simulink model "HW9"  (R2023b)
settings: Solver=FixedStepAuto  StartTime=0.0  StopTime=0.5  FixedStep=0.01  RelTol=1e-3
libraries: simulink_extras x3, sharedtransform x1, uavutilslib x1
settings Model: Creator=Bw Jiang  LastModifiedBy=Bw Jiang

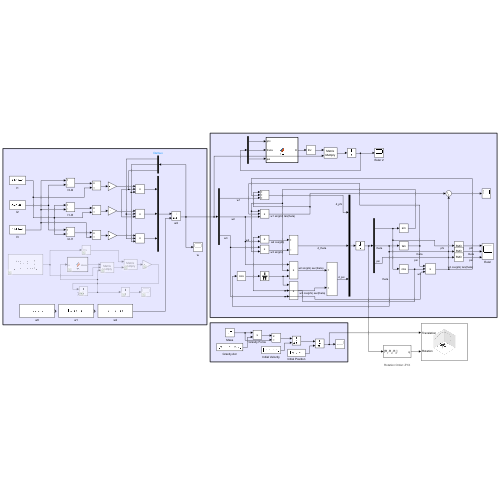
[thumbnail: Simulink's stored preview of the top-level diagram]
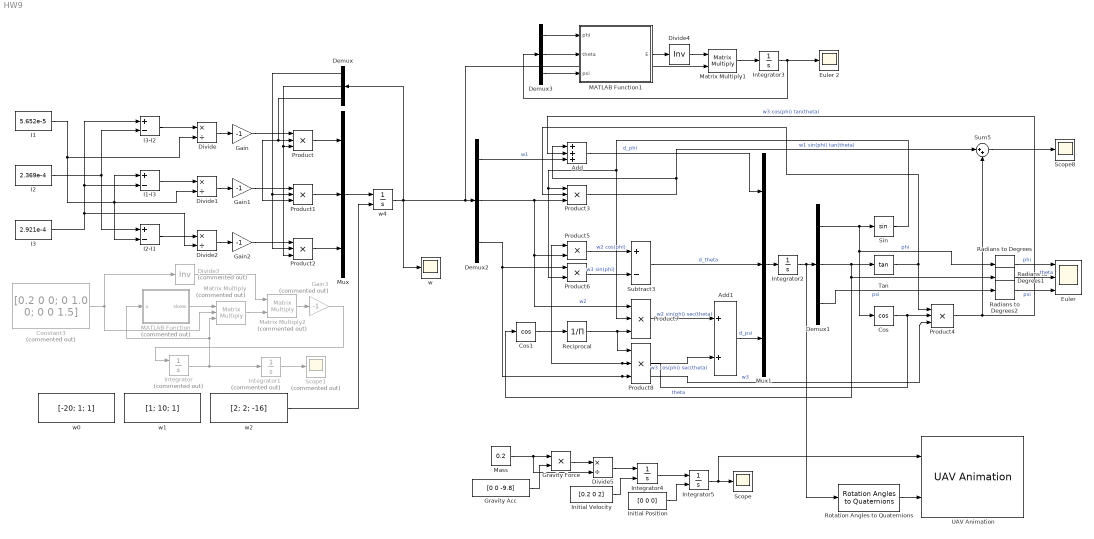
== system HW9 ==
  Add : Sum  Inputs=+++
  Add1 : Sum
  Constant3 : Constant  Commented=on  Value=[0.2 0 0; 0 1.0 0; 0 0 1.5]
  Cos : Trigonometry  Operator=cos
  Cos1 : Trigonometry  Operator=cos
  Demux{,1..3} (4 alike) : Demux  Outputs=3
  Divide{,1..2,5} (4 alike) : Product  Inputs=*/
  Divide3 : Product  Commented=on  Inputs=/  Multiplication=Matrix(*)
  Divide4 : Product  Inputs=/  Multiplication=Matrix(*)
  Euler : Scope  NumInputPorts=3
  Euler 2 : Scope
  Gain : Gain  Gain=-1
  Gain1 : Gain  Gain=-1
  Gain2 : Gain  Gain=-1
  Gain3 : Gain  Commented=on  Gain=-1
  Gravity Acc : Constant  Value=[0 0 -9.8]
  Gravity Force : Product
  I1 : Constant  Value=5.652e-5
  I1-I3 : Sum  Inputs=+-
  I2 : Constant  Value=2.369e-4
  I2-I1 : Sum  Inputs=+-
  I3 : Constant  Value=2.921e-4
  I3-I2 : Sum  Inputs=+-
  Initial Position : Constant  Value=[0 0 0]
  Initial Velocity : Constant  Value=[0.2 0 2]
  Integrator : Integrator  Commented=on  InitialConditionSource=external
  Integrator1 : Integrator  Commented=on
  Integrator2 : Integrator
  Integrator3 : Integrator
  Integrator4 : Integrator  InitialConditionSource=external
  Integrator5 : Integrator  InitialConditionSource=external
  MATLAB Function : MATLAB Function  Commented=on  TreatAsAtomicUnit=on
  MATLAB Function1 : MATLAB Function  TreatAsAtomicUnit=on
  Mass : Constant  Value=0.2
  Matrix Multiply : Product  Commented=on  Inputs=3  Multiplication=Matrix(*)
  Matrix Multiply1 : Product  Multiplication=Matrix(*)
  Matrix Multiply2 : Product  Commented=on  Multiplication=Matrix(*)
  Mux : Mux  Inputs=3
  Mux1 : Mux  Inputs=3
  Product{,1..4,7..8} (7 alike) : Product  Inputs=3
  Product5 : Product
  Product6 : Product
  Radians to Degrees : simulink_extras/Transformations/Radians to Degrees
  Radians to Degrees1 : simulink_extras/Transformations/Radians to Degrees
  Radians to Degrees2 : simulink_extras/Transformations/Radians to Degrees
  Reciprocal : Product  Inputs=/
  Rotation Angles to Quaternions : sharedtransform/Rotation Angles to Quaternions  rotationOrder=ZYX  aMode=aMode
  Scope : Scope
  Scope1 : Scope  Commented=on
  Scope8 : Scope
  Sin : Trigonometry
  Subtract3 : Sum  Inputs=+-
  Sum5 : Sum  Inputs=|++
  Tan : Trigonometry  Operator=tan
  UAV Animation : uavutilslib/UAV Animation  UAVType=FixedWing  UAVSize=0.1  InertialZDirection=Up  SampleTime=-1
  w : Scope
  w0 : Constant  Value=[-20; 1; 1]
  w1 : Constant  Value=[1; 10; 1]
  w2 : Constant  Value=[2; 2; -16]
  w4 : Integrator  InitialConditionSource=external
  wires:
  I3/1 -> Divide2/2, I3-I2/1, I1-I3/2
  I2/1 -> I2-I1/1, I3-I2/2
  I1/1 -> Divide1/2, I2-I1/2, I1-I3/1, Divide/2
  I3-I2/1 -> Divide/1
  I1-I3/1 -> Divide1/1
  I2-I1/1 -> Divide2/1
  Divide/1 -> Gain/1
  Divide2/1 -> Gain2/1
  Divide1/1 -> Gain1/1
  Gain/1 -> Product/1
  Gain1/1 -> Product1/1
  Product1/1 -> Mux/2
  Gain2/1 -> Product2/1
  Product2/1 -> Mux/3
  Product/1 -> Mux/1
  Constant3/1 -> Divide3/1, Matrix Multiply/2
  w2/1 -> w4/2
  Integrator/1 -> Integrator1/1, Matrix Multiply/3, MATLAB Function/1(u)
  MATLAB Function/1(skew) -> Matrix Multiply/1
  Divide3/1 -> Matrix Multiply2/1
  Matrix Multiply/1 -> Matrix Multiply2/2
  Matrix Multiply2/1 -> Gain3/1
  Gain3/1 -> Integrator/1
  Integrator1/1 -> Scope1/1
  Subtract3/1 -> Mux1/2  "d_theta"
  Demux1/3 -> Radians to Degrees2/1  "psi"
  Demux1/2 -> Tan/1, Cos1/1, Radians to Degrees1/1  "theta"
  Product3/1 -> Sum5/1, Add/1  "w1 sin(phi) tan(theta)"
  Product8/1 -> Add1/2  "w3 cos(phi) sec(theta)"
  Demux2/3 -> Product6/1, Product8/3, Product4/3  "w3"
  Add1/1 -> Mux1/3  "d_psi"
  Sum5/1 -> Scope8/1
  Product7/1 -> Add1/1  "w2 sin(phi) sec(theta)"
  Reciprocal/1 -> Product7/3, Product8/1
  Product5/1 -> Subtract3/1  "w2 cos(phi)"
  Cos1/1 -> Reciprocal/1
  Cos/1 -> Product4/2, Product5/1, Product8/2
  Demux1/1 -> Sin/1, Radians to Degrees/1, Cos/1  "phi"
  Tan/1 -> Product4/1, Product3/2
  Product4/1 -> Add/2, Sum5/2  "w3 cos(phi) tan(theta)"
  Demux2/2 -> Product5/2, Product7/1, Product3/3  "w2"
  Integrator2/1 -> Rotation Angles to Quaternions/1, Demux1/1
  Sin/1 -> Product6/2, Product3/1, Product7/2
  Mux1/1 -> Integrator2/1
  Demux2/1 -> Add/3  "w1"
  Product6/1 -> Subtract3/2  "w3 sin(phi)"
  Add/1 -> Mux1/1  "d_phi"
  Radians to Degrees/1 -> Euler/1  "phi"
  Radians to Degrees1/1 -> Euler/2  "theta"
  Radians to Degrees2/1 -> Euler/3  "psi"
  Mux/1 -> w4/1
  Demux/1 -> Product2/2, Product1/2
  Demux/2 -> Product2/3, Product/3
  Demux/3 -> Product/2, Product1/3
  MATLAB Function1/1(E) -> Divide4/1
  Divide4/1 -> Matrix Multiply1/1
  w4/1 -> Matrix Multiply1/2, Demux2/1, w/1, Demux/1
  Matrix Multiply1/1 -> Integrator3/1
  Demux3/2 -> MATLAB Function1/2(theta)
  Demux3/1 -> MATLAB Function1/1(phi)
  Demux3/3 -> MATLAB Function1/3(psi)
  Integrator3/1 -> Euler 2/1, Demux3/1
  Initial Velocity/1 -> Integrator4/2
  Gravity Acc/1 -> Gravity Force/2
  Divide5/1 -> Integrator4/1
  Integrator4/1 -> Integrator5/1
  Initial Position/1 -> Integrator5/2
  Integrator5/1 -> Scope/1, UAV Animation/1
  Mass/1 -> Gravity Force/1, Divide5/2
  Gravity Force/1 -> Divide5/1
  Rotation Angles to Quaternions/1 -> UAV Animation/2

== matlab function HW9/MATLAB Function ==
  data: u input; skew output
function skew = fcn(u)

u1 = u(1);
u2 = u(2);
u3 = u(3);

skew = [0 -u3, u2;
        u3, 0, -u1;
        -u2, u1, 0];

end

== matlab function HW9/MATLAB Function1 ==
  data: phi input; E output; theta input; psi input
function E = fcn(phi, theta, psi)

E = [1, 0, sin(phi);
    0, cos(phi), cos(theta) * sin(phi);
    0, -sin(phi), cos(theta) * cos(phi)];

end
